simulink model "lqr_sim"  (R2025b)
settings: Solver=VariableStepAuto  StartTime=0.0  StopTime=Tfin  RelTol=1e-3
values from neighbouring files (symbols this model uses):
  D1 = K(2)    [lqr_track.m]
  D2 = K(4)    [lqr_track.m]
  E = [0 ... (first row only)    [lqr_track.m]
  F = A - B*K    [lqr_track.m]
  K = lqr(A, B, Q, R)    [lqr_track.m]
  N1 = 10 / tau_d1    [lqr_track.m]
  N2 = 10 / tau_d2    [lqr_track.m]
  P1 = K(1)    [lqr_track.m]
  P2 = K(3)    [lqr_track.m]
  refPoses = [Xr, Yr, psir]    [PID_Stanley_track.m]    (also in lqr_track.m)
  ze0 = [X0; Y0; psi0; vx0; vy0; wpsi0]    [lqr_track.m]
libraries: slpidlib x2
settings Model: Creator=denni  LastModifiedBy=denni

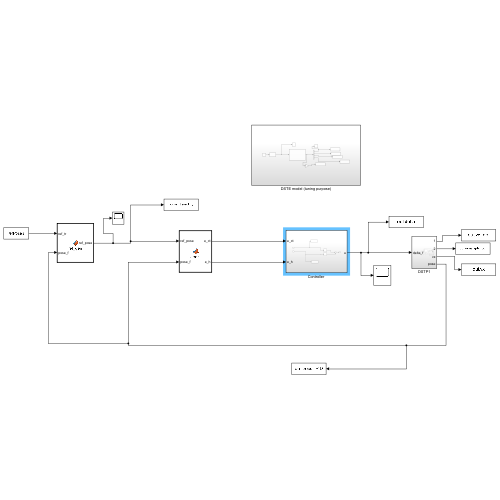
[thumbnail: Simulink's stored preview of the top-level diagram]
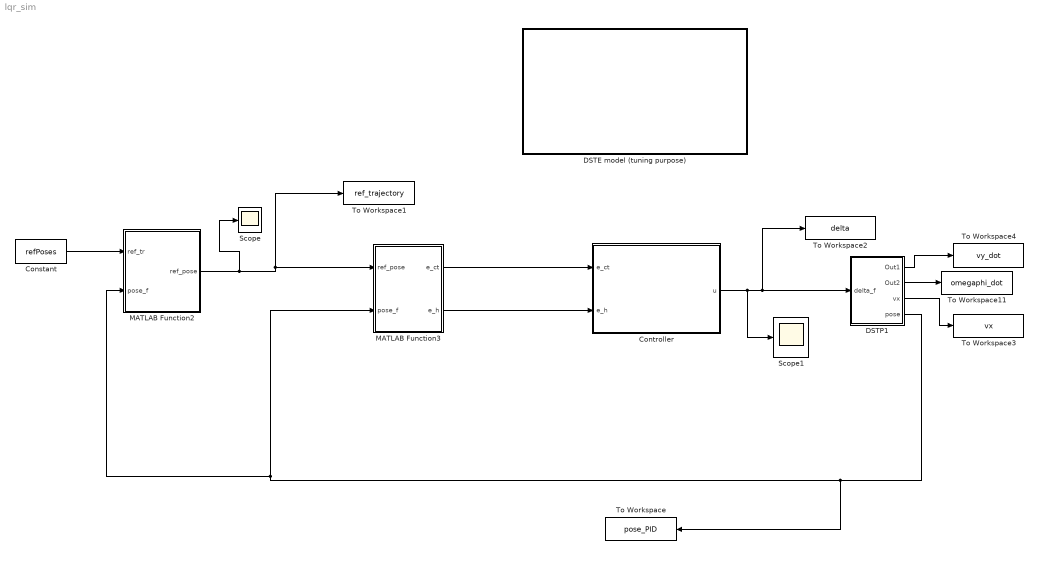
== system lqr_sim ==
  Constant : Constant  Value=refPoses
  "Controller " : Subsystem
  DSTE model (tuning purpose) : Subsystem
  DSTP1 : Subsystem
  MATLAB Function2 : MATLAB Function  TreatAsAtomicUnit=on
  MATLAB Function3 : MATLAB Function  TreatAsAtomicUnit=on  VariantControl=Choice
  Scope : Scope
      settings: ActiveDisplayYMinimum=-63.55901895753157  ActiveDisplayYMaximum=93.327516738493628  DataLoggingVariableName=ScopeData3
  Scope1 : Scope
      settings: ActiveDisplayYMinimum=-1  ActiveDisplayYMaximum=1  DataLoggingVariableName=ScopeData2
  To Workspace : ToWorkspace  VariableName=pose_PID  SaveFormat=Timeseries  SampleTime=-1
  To Workspace1 : ToWorkspace  VariableName=ref_trajectory  SaveFormat=Timeseries  SampleTime=-1
  To Workspace11 : ToWorkspace  VariableName=omegaphi_dot  SaveFormat=Timeseries  SampleTime=-1
      settings: Save2DSignal=2-D array (concatenate along first dimension)
  To Workspace2 : ToWorkspace  VariableName=delta  SaveFormat=Timeseries  SampleTime=-1
  To Workspace3 : ToWorkspace  VariableName=vx  SaveFormat=Timeseries  SampleTime=-1
      settings: Save2DSignal=2-D array (concatenate along first dimension)
  To Workspace4 : ToWorkspace  VariableName=vy_dot  SaveFormat=Timeseries  SampleTime=-1
      settings: Save2DSignal=2-D array (concatenate along first dimension)
  wires:
  MATLAB Function3/2(e_h) -> "Controller "/2(e_h)
  Constant/1 -> MATLAB Function2/1(ref_tr)
  MATLAB Function2/1(ref_pose) -> Scope/1, To Workspace1/1, MATLAB Function3/1(ref_pose)
  DSTP1/4(pose) -> To Workspace/1, MATLAB Function3/2(pose_f), MATLAB Function2/2(pose_f)
  DSTP1/1(Out1) -> To Workspace4/1
  DSTP1/3(vx) -> To Workspace3/1
  DSTP1/2(Out2) -> To Workspace11/1
  MATLAB Function3/1(e_ct) -> "Controller "/1(e_ct)
  "Controller "/1(u) -> Scope1/1, DSTP1/1(delta_f), To Workspace2/1

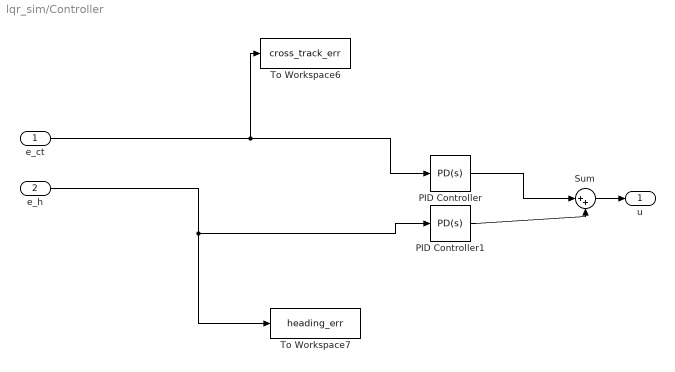
== system lqr_sim/Controller  ==
  e_ct : Inport
  e_h : Inport  Port=2
  PID Controller : slpidlib/PID Controller  Controller=PD  Form=Parallel  TimeDomain=Continuous-time  UseExternalTs=off  SampleTime=-1  IntegratorMethod=Forward Euler  FilterMethod=Forward Euler  ControllerParametersSource=internal  P=P1  I=1  UseKiTs=off  D=D1  UseExternalDerivativeSource=off  N=N1  UseFilter=on  TunerSelectOption=Transfer Function Based (PID Tuner App)  InitialConditionSource=internal  InitialConditionForIntegrator=0  InitialConditionForFilter=0  DifferentiatorICPrevScaledInput=0  ExternalReset=none  TrackingMode=off  Kt=1  LimitOutput=off  SatLimitsSource=internal  UpperSaturationLimit=inf  LowerSaturationLimit=-inf  LinearizeAsGain=on  AntiWindupMode=none  Kb=1  LimitIntegrator=off  UpperIntegratorSaturationLimit=inf  LowerIntegratorSaturationLimit=-inf  POutMin=[]  POutMax=[]  IOutMin=[]  IOutMax=[]  DOutMin=[]  DOutMax=[]  NOutMin=[]  NOutMax=[]  SumOutMin=[]  SumOutMax=[]  SaturationOutMin=[]  SaturationOutMax=[]  PParamMin=[]  PParamMax=[]  IParamMin=[]  IParamMax=[]  DParamMin=[]  DParamMax=[]  NParamMin=[]  NParamMax=[]  KbParamMin=[]  KbParamMax=[]  KtParamMin=[]  KtParamMax=[]  KbOutMin=[]  KbOutMax=[]  KtOutMin=[]  KtOutMax=[]  IntegratorOutMin=[]  IntegratorOutMax=[]  FilterOutMin=[]  FilterOutMax=[]  SumI1OutMin=[]  SumI1OutMax=[]  SumI2OutMin=[]  SumI2OutMax=[]  SumI3OutMin=[]  SumI3OutMax=[]  SumI4OutMin=[]  SumI4OutMax=[]  SumDOutMin=[]  SumDOutMax=[]  DifferentiatorOutMin=[]  DifferentiatorOutMax=[]  FilterDiffOutCoefMin=[]  FilterDiffOutCoefMax=[]  ReciprocalOutMin=[]  ReciprocalOutMax=[]  SumDenOutMin=[]  SumDenOutMax=[]  SumNumOutMin=[]  SumNumOutMax=[]  DivideOutMin=[]  DivideOutMax=[]  UdiffTsProdOutMin=[]  UdiffTsProdOutMax=[]  NTsProdOutMin=[]  NTsProdOutMax=[]  UintegralTsProdOutMin=[]  UintegralTsProdOutMax=[]  UngainTsProdOutMin=[]  UngainTsProdOutMax=[]  ClampingZeroOutDataTypeStr=Inherit: Inherit via back propagation  ClampingZeroOutMin=[]  ClampingZeroOutMax=[]  FilterDenConstantOutDataTypeStr=Inherit: Inherit via back propagation  FilterDenConstantOutMin=[]  FilterDenConstantOutMax=[]  PCopyOutDataTypeStr=Inherit: Inherit via back propagation  PCopyOutMin=[]  PCopyOutMax=[]  NCopyOutDataTypeStr=Inherit: Inherit via back propagation  NCopyOutMin=[]  NCopyOutMax=[]  IntegratorContinuousStateAttributes=''  IntegratorStateMustResolveToSignalObject=off  IntegratorRTWStateStorageClass=Auto  FilterContinuousStateAttributes=''  FilterStateMustResolveToSignalObject=off  FilterRTWStateStorageClass=Auto  ParallelPVariant=InternalParameters  IdealPVariant=Disabled  IVariant=Disabled  DVariant=InternalParameters  IntegratorVariant=Disabled  SatVariant=Disabled  AWVariant=Disabled  PCopyVariant=Disabled  TRVariant=Disabled  FdbkBlocksVariant=Forward  IdealPFdbkVariant=Disabled  SatFdbkVariant=Disabled  DerivativeFilterVariant=ContFilter  NVariant=InternalParameters  NCopyVariant=Disabled  FilterICVariant=InternalICsFilter  IntegratorICVariant=Disabled  ExternalResetVariant=Disabled  TRSumVariant=Passthrough  SumFdbkVariant=Disabled  SumVariant=Sum_PD  TsampFilterVariant=InternalTs  TsampNgainVariant=Passthrough  TsampIntegralVariant=Disabled_SignalSpec  ExternalSaturationOutDataTypeStr=Inherit: Same as second input  DerivativeSourceVariant=ErrorSignal  PreIntVariant=InternalPreInt
  PID Controller1 : slpidlib/PID Controller  Controller=PD  Form=Parallel  TimeDomain=Continuous-time  UseExternalTs=off  SampleTime=-1  IntegratorMethod=Forward Euler  FilterMethod=Forward Euler  ControllerParametersSource=internal  P=P2  I=1  UseKiTs=off  D=D2  UseExternalDerivativeSource=off  N=N2  UseFilter=on  TunerSelectOption=Transfer Function Based (PID Tuner App)  InitialConditionSource=internal  InitialConditionForIntegrator=0  InitialConditionForFilter=0  DifferentiatorICPrevScaledInput=0  ExternalReset=none  TrackingMode=off  Kt=1  LimitOutput=off  SatLimitsSource=internal  UpperSaturationLimit=inf  LowerSaturationLimit=-inf  LinearizeAsGain=on  AntiWindupMode=none  Kb=1  LimitIntegrator=off  UpperIntegratorSaturationLimit=inf  LowerIntegratorSaturationLimit=-inf  POutMin=[]  POutMax=[]  IOutMin=[]  IOutMax=[]  DOutMin=[]  DOutMax=[]  NOutMin=[]  NOutMax=[]  SumOutMin=[]  SumOutMax=[]  SaturationOutMin=[]  SaturationOutMax=[]  PParamMin=[]  PParamMax=[]  IParamMin=[]  IParamMax=[]  DParamMin=[]  DParamMax=[]  NParamMin=[]  NParamMax=[]  KbParamMin=[]  KbParamMax=[]  KtParamMin=[]  KtParamMax=[]  KbOutMin=[]  KbOutMax=[]  KtOutMin=[]  KtOutMax=[]  IntegratorOutMin=[]  IntegratorOutMax=[]  FilterOutMin=[]  FilterOutMax=[]  SumI1OutMin=[]  SumI1OutMax=[]  SumI2OutMin=[]  SumI2OutMax=[]  SumI3OutMin=[]  SumI3OutMax=[]  SumI4OutMin=[]  SumI4OutMax=[]  SumDOutMin=[]  SumDOutMax=[]  DifferentiatorOutMin=[]  DifferentiatorOutMax=[]  FilterDiffOutCoefMin=[]  FilterDiffOutCoefMax=[]  ReciprocalOutMin=[]  ReciprocalOutMax=[]  SumDenOutMin=[]  SumDenOutMax=[]  SumNumOutMin=[]  SumNumOutMax=[]  DivideOutMin=[]  DivideOutMax=[]  UdiffTsProdOutMin=[]  UdiffTsProdOutMax=[]  NTsProdOutMin=[]  NTsProdOutMax=[]  UintegralTsProdOutMin=[]  UintegralTsProdOutMax=[]  UngainTsProdOutMin=[]  UngainTsProdOutMax=[]  ClampingZeroOutDataTypeStr=Inherit: Inherit via back propagation  ClampingZeroOutMin=[]  ClampingZeroOutMax=[]  FilterDenConstantOutDataTypeStr=Inherit: Inherit via back propagation  FilterDenConstantOutMin=[]  FilterDenConstantOutMax=[]  PCopyOutDataTypeStr=Inherit: Inherit via back propagation  PCopyOutMin=[]  PCopyOutMax=[]  NCopyOutDataTypeStr=Inherit: Inherit via back propagation  NCopyOutMin=[]  NCopyOutMax=[]  IntegratorContinuousStateAttributes=''  IntegratorStateMustResolveToSignalObject=off  IntegratorRTWStateStorageClass=Auto  FilterContinuousStateAttributes=''  FilterStateMustResolveToSignalObject=off  FilterRTWStateStorageClass=Auto  ParallelPVariant=InternalParameters  IdealPVariant=Disabled  IVariant=Disabled  DVariant=InternalParameters  IntegratorVariant=Disabled  SatVariant=Disabled  AWVariant=Disabled  PCopyVariant=Disabled  TRVariant=Disabled  FdbkBlocksVariant=Forward  IdealPFdbkVariant=Disabled  SatFdbkVariant=Disabled  DerivativeFilterVariant=ContFilter  NVariant=InternalParameters  NCopyVariant=Disabled  FilterICVariant=InternalICsFilter  IntegratorICVariant=Disabled  ExternalResetVariant=Disabled  TRSumVariant=Passthrough  SumFdbkVariant=Disabled  SumVariant=Sum_PD  TsampFilterVariant=InternalTs  TsampNgainVariant=Passthrough  TsampIntegralVariant=Disabled_SignalSpec  ExternalSaturationOutDataTypeStr=Inherit: Same as second input  DerivativeSourceVariant=ErrorSignal  PreIntVariant=InternalPreInt
  Sum : Sum  Inputs=|++
  To Workspace6 : ToWorkspace  VariableName=cross_track_err  SaveFormat=Timeseries  SampleTime=-1
  To Workspace7 : ToWorkspace  VariableName=heading_err  SaveFormat=Timeseries  SampleTime=-1
  u : Outport
  wires:
  e_h/1 -> PID Controller1/1, To Workspace7/1
  e_ct/1 -> PID Controller/1, To Workspace6/1
  PID Controller/1 -> Sum/1
  PID Controller1/1 -> Sum/2
  Sum/1 -> u/1

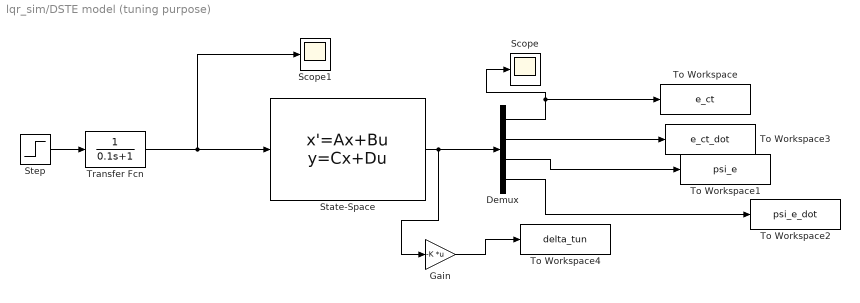
== system lqr_sim/DSTE model (tuning purpose) ==
  Demux : Demux
  Gain : Gain  Gain=-K  Multiplication=Matrix(K*u)
  Scope : Scope
      settings: ActiveDisplayYMinimum=-1  ActiveDisplayYMaximum=1
  Scope1 : Scope
      settings: ActiveDisplayYMinimum=-5.438579112963331  ActiveDisplayYMaximum=1.036380233363509
  State-Space : StateSpace  A=F  B=E  C=eye(4)  D=zeros(4,1)  InitialCondition=0  AllowTunableDMatrix=on
  Step : Step  After=1*pi/180  SampleTime=0
  To Workspace : ToWorkspace  VariableName=e_ct  SaveFormat=Timeseries  SampleTime=-1
  To Workspace1 : ToWorkspace  VariableName=psi_e  SaveFormat=Timeseries  SampleTime=-1
  To Workspace2 : ToWorkspace  VariableName=psi_e_dot  SaveFormat=Timeseries  SampleTime=-1
  To Workspace3 : ToWorkspace  VariableName=e_ct_dot  SaveFormat=Timeseries  SampleTime=-1
  To Workspace4 : ToWorkspace  VariableName=delta_tun  SaveFormat=Timeseries  SampleTime=-1
  Transfer Fcn : TransferFcn  Denominator=[0.1 1]
  wires:
  Demux/4 -> To Workspace2/1
  Step/1 -> Transfer Fcn/1
  State-Space/1 -> Demux/1, Gain/1
  Demux/1 -> Scope/1, To Workspace/1
  Demux/2 -> To Workspace3/1
  Demux/3 -> To Workspace1/1
  Gain/1 -> To Workspace4/1
  Transfer Fcn/1 -> State-Space/1, Scope1/1

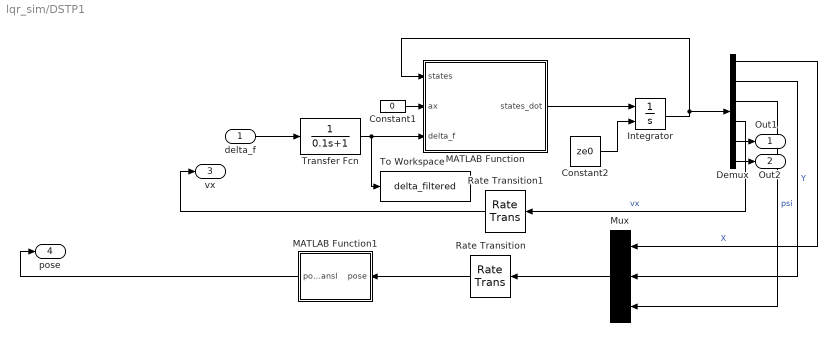
== system lqr_sim/DSTP1 ==
  delta_f : Inport
  Constant1 : Constant  Value=0
  Constant2 : Constant  Value=ze0
  Demux : Demux  Outputs=6
  Integrator : Integrator  InitialConditionSource=external
  MATLAB Function : MATLAB Function  TreatAsAtomicUnit=on
  MATLAB Function1 : MATLAB Function  TreatAsAtomicUnit=on
  Mux : Mux  Inputs=3
  Rate Transition : RateTransition  Deterministic=off
  Rate Transition1 : RateTransition
  To Workspace : ToWorkspace  VariableName=delta_filtered  SaveFormat=Timeseries  SampleTime=-1
  Transfer Fcn : TransferFcn  Denominator=[0.1 1]
  Out1 : Outport
  Out2 : Outport  Port=2
  vx : Outport  Port=3
  pose : Outport  Port=4
  wires:
  Demux/1 -> Mux/1  "X"
  Constant1/1 -> MATLAB Function/2(ax)
  Integrator/1 -> MATLAB Function/1(states), Demux/1
  MATLAB Function/1(states_dot) -> Integrator/1
  Demux/6 -> Out2/1
  Demux/3 -> Mux/3  "psi"
  Transfer Fcn/1 -> To Workspace/1, MATLAB Function/3(delta_f)
  Demux/2 -> Mux/2  "Y"
  Constant2/1 -> Integrator/2
  Demux/5 -> Out1/1
  delta_f/1 -> Transfer Fcn/1
  MATLAB Function1/1(pose_transl) -> pose/1
  Mux/1 -> Rate Transition/1
  Rate Transition/1 -> MATLAB Function1/1(pose)
  Demux/4 -> Rate Transition1/1  "vx"
  Rate Transition1/1 -> vx/1

== matlab function lqr_sim/DSTP1/MATLAB Function ==
  data: states input; states_dot output; ax input; delta_f input
function states_dot  = DST(states, ax, delta_f)

    % Vehicle Parameters
    
    l1 = 1.2;  % Front axle-c.o.g. distance (m)
    l2 = 1.6;  % Rear axle-c.o.g. distance (m)
    m = 1575;   % Vehicle mass (kg)
    Jz = 4000;  % Yaw inertia (kg*m^2))
    
    % Tire parameters
    C1 = 27e3;  % Front tire stiffness
    C2 = C1;    % Rear tire stiffness
    p1 = 3863;
    p2 = 1.5;
    p4 = -0.5;
    p3_f = C1/p1/p2;
    p3_r = C2/p1/p2;
    
    % STATES:
    X = states(1);      % [m]     global X position
    Y = states(2) ;     % [m]     global Y position
    psi =states(3);    % [rad]   yaw angle
    vx = states(4);     % [m/s]   longitudinal velocity (vehicle frame)
    vy = states(5);     % [m/s]   lateral velocity (vehicle frame)
    wpsi = states(6);   % [rad/s] yaw rate
    
    %% Slip angles
    
    alpha1 = atan((vy + l1*wpsi)/vx) - delta_f;
    alpha2 = atan((vy - l2*wpsi)/vx);
     
    %% Pacejka's tyre forces 
    f1 = pacejka_magic (alpha1, p3_f);
    f2 = pacejka_magic (alpha2, p3_r);
    Fy1 = -f1 * cos(delta_f);
    Fy2 = -f2;

    %% State derivatives 
    Xdot    = vx * cos(psi) - vy * sin(psi);
    Ydot    = vx * sin(psi) + vy * cos(psi);
    psidot  = wpsi;
    vxdot   = vy * wpsi + ax;
    vydot   = -vx * wpsi + (2/m)  * (Fy1 + Fy2);
    wpsidot = (2/Jz) * (l1 * Fy1 - l2 * Fy2);
    
    %% Output
    states_dot = [Xdot; Ydot; psidot; vxdot; vydot; wpsidot];
end 

function f = pacejka_magic (alpha, p3)
    p1 = 3863;
    p2 = 1.5;
    p4 = -0.5;
    f = p1 * sin(p2 * atan(p3 * alpha - p4 *(p3 * alpha - atan(p3 * alpha))));
end

== matlab function lqr_sim/DSTP1/MATLAB Function1 ==
  data: pose input; pose_transl output
function pose_transl = TranslatePose(pose)

% Parameters
l1 = 1.2;  % frontal COG distance
X_cog = pose(1);
Y_cog = pose(2);
psi_cog = pose(3);

X_f = X_cog + l1 * cos(psi_cog);
Y_f = Y_cog + l1 * sin(psi_cog);
psi_f = psi_cog;
pose_transl= [X_f;Y_f;psi_f];

== matlab function lqr_sim/MATLAB Function2 ==
  data: ref_tr input; ref_pose output; pose_f input
function ref_pose=ref_gen(ref_tr,pose_f)

N=size(ref_tr,1);

% reference trajectory closest point to the vehicle
dis=vecnorm(ref_tr(:,1:2)'-pose_f(1:2)*ones(1,N));
[~,c]=min(dis);
ref_pose=ref_tr(c,:)';

end

== matlab function lqr_sim/MATLAB Function3 ==
  data: ref_pose input; e_ct output; pose_f input; e_h output
function [e_ct,e_h]=errors(ref_pose,pose_f)

% Wrap angles in the interval [0,2*pi]
ref_pose(3)=wrap_to_2pi(ref_pose(3));
pose_f(3)=wrap_to_2pi(pose_f(3));

% Cross-track error  
d=ref_pose(1:2)-pose_f(1:2);
e_ct=d(2)*cos(ref_pose(3))-d(1)*sin(ref_pose(3));

% Heading error
e_h=wrap_to_pi(ref_pose(3)-pose_f(3));

end

%--------------------------------------------------------------------------

function lambda = wrap_to_2pi(lambda)
%   Wraps angle in radians to [0 2*pi]
%   lambdaWrapped = wrapTo2Pi(LAMBDA) wraps angles in LAMBDA, in radians,
%   to the interval [0 2*pi] such that zero maps to zero and 2*pi maps
%   to 2*pi. (In general, positive multiples of 2*pi map to 2*pi and
%   negative multiples of 2*pi map to zero.)
%   See also wrapToPi, wrapTo180, wrapTo360.
positiveInput = (lambda > 0);
lambda = mod(lambda, 2*pi);
lambda((lambda == 0) & positiveInput) = 2*pi;
end

function lambda = wrap_to_pi(lambda)
%   Wraps angle in radians to [-pi pi]
%   lambdaWrapped = wrapToPi(LAMBDA) wraps angles in LAMBDA, in radians,
%   to the interval [-pi pi] such that pi maps to pi and -pi maps to
%   -pi.  (In general, odd, positive multiples of pi map to pi and odd,
%   negative multiples of pi map to -pi.)
%   See also wrapTo2Pi, wrapTo180, wrapTo360.
q = (lambda < -pi) | (pi < lambda);
lambda(q) = wrap_to_2pi(lambda(q) + pi) - pi;
end
